simulink library "gpkfAltitudeOpt_cl"  (R2020a)
settings: Solver=VariableStepAuto  StartTime=0.0  StopTime=10.0  RelTol=1e-3
undefined symbols (not defined in the file or in its folder): hiLvlCtrl, initializeBussesFromBlock
libraries: dspsigops x3, calculate_vector_magnitude x1, calcKalmanEstimate_ul x1, optimizeAltitude_ul x1
settings Model: Creator=Ayaz  LastModifiedBy=Ayaz

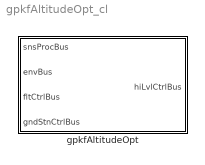
== system gpkfAltitudeOpt_cl ==
  gpkfAltitudeOpt : Subsystem  LoadFcn=initializeBussesFromBlock(gcb)  InitFcn=initializeBussesFromBlock(gcb)  StartFcn=initializeBussesFromBlock(gcb)  mask{hiLvlCtrl=hiLvlCtrl}
      mask prompts: hiLvlCtrl "Hi-level controller object"
      mask TypeOptions hiLvlCtrl: gpkfAltitudeOpt/hiLvlCtrl

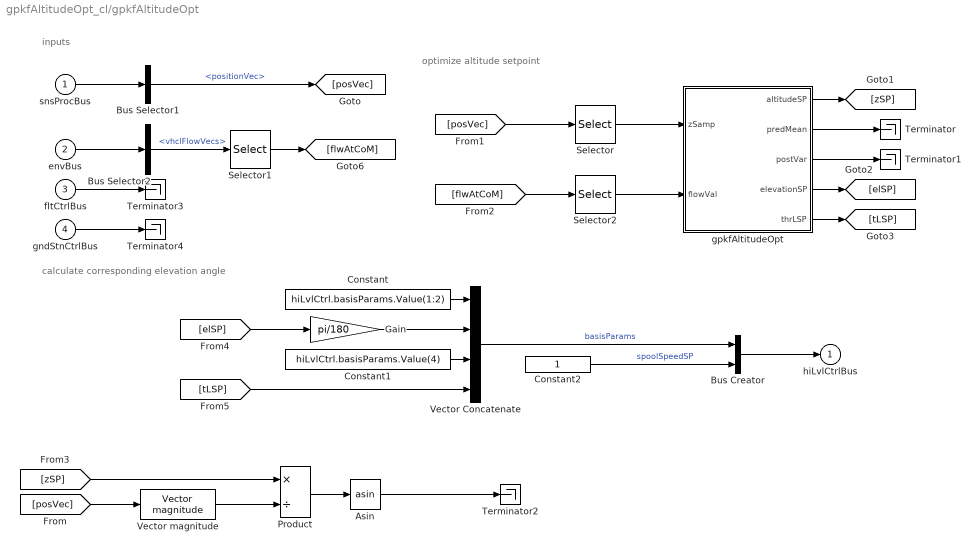
== system gpkfAltitudeOpt_cl/gpkfAltitudeOpt ==
  note: inputs
  note: calculate corresponding elevation angle
  note: optimize altitude setpoint
  snsProcBus : Inport
  envBus : Inport  Port=2
  fltCtrlBus : Inport  Port=3
  gndStnCtrlBus : Inport  Port=4
  Asin : Trigonometry  Operator=asin
  Bus Creator : BusCreator  Inputs=2  OutDataTypeStr=Bus: hiLvlCtrlBus
  Bus Selector1 : BusSelector  OutputSignals=positionVec
  Bus Selector2 : BusSelector  OutputSignals=vhclFlowVecs
  Constant : Constant  Value=hiLvlCtrl.basisParams.Value(1:2)
  Constant1 : Constant  Value=hiLvlCtrl.basisParams.Value(4)
  Constant2 : Constant
  Gain : Gain  Gain=pi/180
  Product : Product  Inputs=*/
  Selector : Selector  NumberOfDimensions=2  InputPortWidth=3  IndexOptions=Index vector (dialog),Index vector (dialog)  Indices=3,1  OutputSizes=1,1
  Selector1 : Selector  NumberOfDimensions=2  InputPortWidth=3  IndexOptions=Select all,Index vector (dialog)  Indices=[1 3],5  OutputSizes=1,1
  Selector2 : Selector  NumberOfDimensions=2  InputPortWidth=3  IndexOptions=Index vector (dialog),Index vector (dialog)  Indices=1,1  OutputSizes=1,1
  Terminator{,1..4} (5 alike) : Terminator
  Vector Concatenate : Concatenate  NumInputs=4
  Vector magnitude : calculate_vector_magnitude/Vector magnitude  SystemSampleTime=-1  Latency=0  AutoFrameSizeCalculation=off
  gpkfAltitudeOpt : Subsystem  mask{hiLvlCtrl=hiLvlCtrl}
      mask prompts: hiLvlCtrl "Hi-level controller object"
      mask TypeOptions hiLvlCtrl: calcKalmanEstimate/hiLvlCtrl | optimizeAltitude/hiLvlCtrl
  hiLvlCtrlBus : Outport
  wires:
  Selector1/1 -> [flwAtCoM]
  [flwAtCoM] -> Selector2/1
  Bus Selector2/1 -> Selector1/1  "<vhclFlowVecs>"
  Selector2/1 -> gpkfAltitudeOpt/2(flowVal)
  Constant1/1 -> Vector Concatenate/3
  Constant/1 -> Vector Concatenate/1
  Vector Concatenate/1 -> Bus Creator/1  "basisParams"
  [posVec] -> Selector/1
  Selector/1 -> gpkfAltitudeOpt/1(zSamp)
  gpkfAltitudeOpt/1(altitudeSP) -> [zSP]
  Vector magnitude/1 -> Product/2
  [posVec] -> Vector magnitude/1
  gpkfAltitudeOpt/2(predMean) -> Terminator/1
  fltCtrlBus/1 -> Terminator3/1
  snsProcBus/1 -> Bus Selector1/1
  Bus Selector1/1 -> [posVec]  "<positionVec>"
  envBus/1 -> Bus Selector2/1
  Bus Creator/1 -> hiLvlCtrlBus/1
  gpkfAltitudeOpt/3(postVar) -> Terminator1/1
  gndStnCtrlBus/1 -> Terminator4/1
  [zSP] -> Product/1
  Product/1 -> Asin/1
  Asin/1 -> Terminator2/1
  gpkfAltitudeOpt/5(thrLSP) -> [tLSP]
  gpkfAltitudeOpt/4(elevationSP) -> [elSP]
  [elSP] -> Gain/1
  Gain/1 -> Vector Concatenate/2
  [tLSP] -> Vector Concatenate/4
  Constant2/1 -> Bus Creator/2  "spoolSpeedSP"

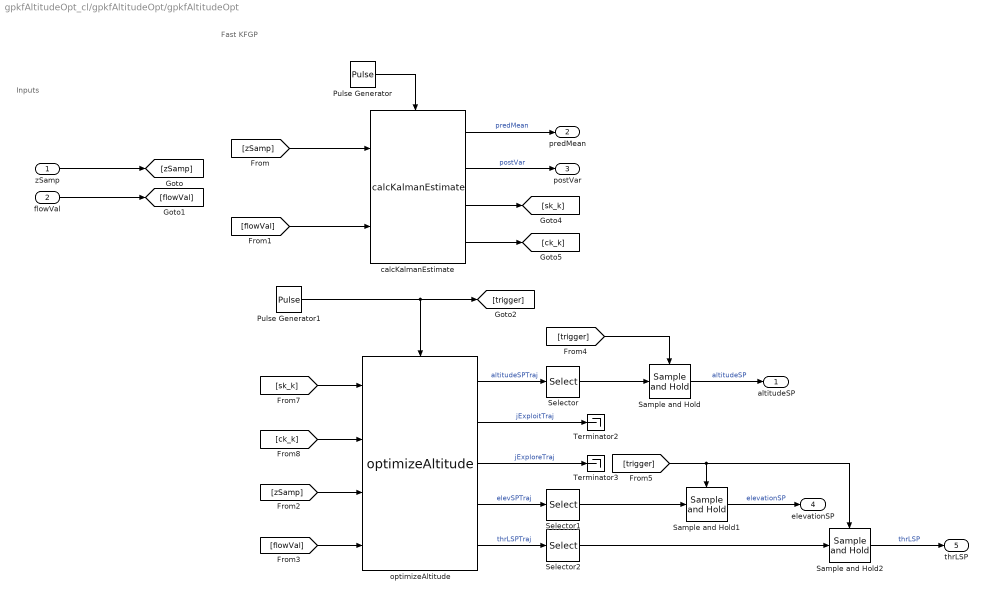
== system gpkfAltitudeOpt_cl/gpkfAltitudeOpt/gpkfAltitudeOpt ==
  note: Fast KFGP
  note: Inputs
  zSamp : Inport
  flowVal : Inport  Port=2
  Pulse Generator : DiscretePulseGenerator  PulseType=Time based  Period=hiLvlCtrl.kfgpTimeStep*60
  Pulse Generator1 : DiscretePulseGenerator  PulseType=Time based  Period=hiLvlCtrl.mpckfgpTimeStep*60  PhaseDelay=hiLvlCtrl.mpckfgpTimeStep*60
  Sample and Hold : dspsigops/Sample and Hold  trig=Rising edge  initCond=hiLvlCtrl.initVals(1)  latchinput=off
  Sample and Hold1 : dspsigops/Sample and Hold  trig=Rising edge  initCond=hiLvlCtrl.initVals(2)  latchinput=off
  Sample and Hold2 : dspsigops/Sample and Hold  trig=Rising edge  initCond=hiLvlCtrl.initVals(3)  latchinput=off
  Selector : Selector  InputPortWidth=hiLvlCtrl.predictionHorz  IndexOptions=Index vector (dialog)  Indices=1  OutputSizes=1
  Selector1 : Selector  InputPortWidth=hiLvlCtrl.predictionHorz  IndexOptions=Index vector (dialog)  Indices=1  OutputSizes=1
  Selector2 : Selector  InputPortWidth=hiLvlCtrl.predictionHorz  IndexOptions=Index vector (dialog)  Indices=1  OutputSizes=1
  Terminator2 : Terminator
  Terminator3 : Terminator
  calcKalmanEstimate : calcKalmanEstimate_ul/calcKalmanEstimate  hiLvlCtrl=hiLvlCtrl
  optimizeAltitude : optimizeAltitude_ul/optimizeAltitude  hiLvlCtrl=hiLvlCtrl
  altitudeSP : Outport
  predMean : Outport  Port=2
  postVar : Outport  Port=3
  elevationSP : Outport  Port=4
  thrLSP : Outport  Port=5
  wires:
  calcKalmanEstimate/3 -> [sk_k]
  calcKalmanEstimate/4 -> [ck_k]
  flowVal/1 -> [flowVal]
  zSamp/1 -> [zSamp]
  [zSamp] -> calcKalmanEstimate/1
  [flowVal] -> calcKalmanEstimate/2
  [zSamp] -> optimizeAltitude/3
  calcKalmanEstimate/1 -> predMean/1  "predMean"
  calcKalmanEstimate/2 -> postVar/1  "postVar"
  optimizeAltitude/2 -> Terminator2/1  "jExploitTraj"
  optimizeAltitude/3 -> Terminator3/1  "jExploreTraj"
  Sample and Hold/1 -> altitudeSP/1  "altitudeSP"
  Pulse Generator/1 -> calcKalmanEstimate/Trigger
  Pulse Generator1/1 -> optimizeAltitude/Trigger, [trigger]
  optimizeAltitude/1 -> Selector/1  "altitudeSPTraj"
  [sk_k] -> optimizeAltitude/1
  [ck_k] -> optimizeAltitude/2
  [flowVal] -> optimizeAltitude/4
  Selector/1 -> Sample and Hold/1
  Selector1/1 -> Sample and Hold1/1
  Sample and Hold1/1 -> elevationSP/1  "elevationSP"
  optimizeAltitude/4 -> Selector1/1  "elevSPTraj"
  Selector2/1 -> Sample and Hold2/1
  Sample and Hold2/1 -> thrLSP/1  "thrLSP"
  optimizeAltitude/5 -> Selector2/1  "thrLSPTraj"
  [trigger] -> Sample and Hold/Trigger
  [trigger] -> Sample and Hold2/Trigger, Sample and Hold1/Trigger
